simulink model "Simulacion_control"  (R2016a)
settings: Solver=ode4  SolverMode=SingleTasking  StartTime=0.0  StopTime=16  FixedStep=0.0001  RelTol=1e-3
undefined symbols (not defined in the file): ADAMS_cwd, ADAMS_exec, ADAMS_host, ADAMS_init, ADAMS_inputs, ADAMS_outputs, ADAMS_prefix, ADAMS_static, ADAMS_sysdir
libraries: simulink x5
settings Model: Creator=JoseSosa  LastModifiedBy=jrsos
settings DebuggingCC: SFUnexpectedBacktrackingDiag=error  SFNoUnconditionalDefaultTransitionDiag=error
settings SFSimCC: SimUseLocalCustomCode=on
settings RTWCC: RTWUseLocalCustomCode=on
settings GRTTargetCC: TargetLangStandard=C99 (ISO)  GeneratePreprocessorConditionals=Use local settings
settings ConfigComp: CovMetricSettings=dwe  CovHtmlReporting=off  CovSaveCumulativeToWorkspaceVar=off  CovSaveSingleToWorkspaceVar=off  CovExternalEMLEnable=on

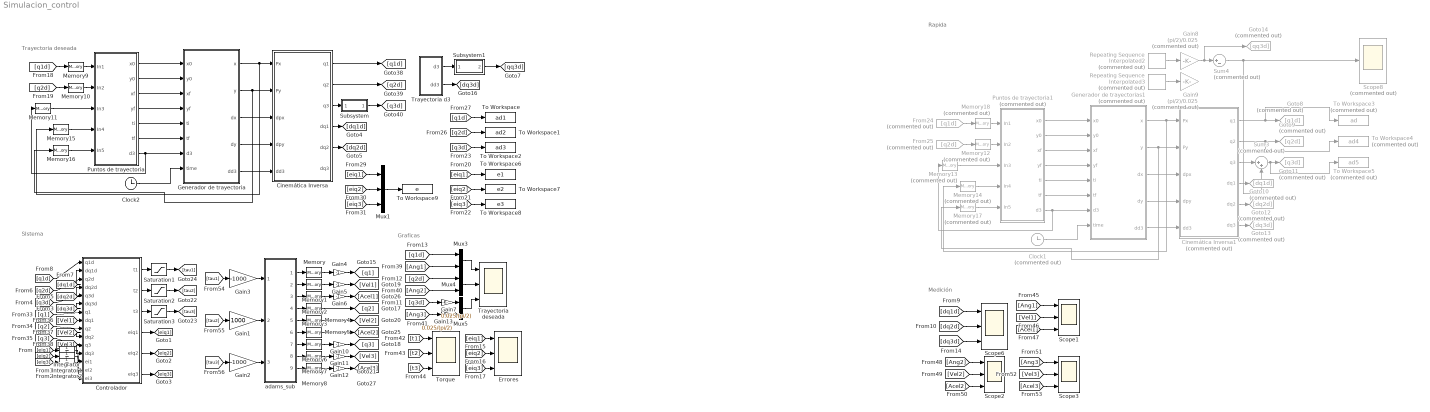
== system Simulacion_control ==
  note: Medición
  note: Graficas
  note: SIstema
  note: Trayectoria deseada
  note: Rapida
  Cinemática Inversa : MATLAB Function  TreatAsAtomicUnit=on
  Cinemática Inversa1 : MATLAB Function  Commented=on  TreatAsAtomicUnit=on
  Clock1 : Clock  Commented=on
  Clock2 : Clock
      settings: Decimation=16
  Controlador : MATLAB Function  TreatAsAtomicUnit=on
  "Errores " : Scope  NumInputPorts=3
  From24 : From  Commented=on  GotoTag=q1d
  From25 : From  Commented=on  GotoTag=q2d
  Gain1 : Gain  Gain=1000
  Gain{4..6,10..12} (6 alike) : Gain  Gain=-1
  Gain13 : Gain  Gain=0.025/(pi/2)
  Gain2 : Gain  Gain=-1000
  Gain3 : Gain  Gain=-1000
  Gain7 : Gain  Gain=0.025/(pi/2)
  Gain8 : Gain  Commented=on  Gain=(pi/2)/0.025
  Gain9 : Gain  Commented=on  Gain=(pi/2)/0.025
  Generador de trayectoria : MATLAB Function  TreatAsAtomicUnit=on
  Generador de trayectorias1 : MATLAB Function  Commented=on  TreatAsAtomicUnit=on
  Goto10 : Goto  Commented=on  GotoTag=dq1d
  Goto11 : Goto  Commented=on  GotoTag=q3d
  Goto12 : Goto  Commented=on  GotoTag=dq2d
  Goto13 : Goto  Commented=on  GotoTag=dq3d
  Goto14 : Goto  Commented=on  GotoTag=qq3d
  Goto8 : Goto  Commented=on  GotoTag=q1d
  Goto9 : Goto  Commented=on  GotoTag=q2d
  Integrator : Integrator
  Integrator1 : Integrator
  Integrator2 : Integrator
  Memory{,1..11,15..16} (14 alike) : Memory
  Memory{12..14,17..18} (5 alike) : Memory  Commented=on
  Mux1 : Mux  Inputs=3
  Mux3 : Mux  Inputs=2
  Mux4 : Mux  Inputs=2
  Mux5 : Mux  Inputs=2
  Puntos de trayectoria : Subsystem
  Puntos de trayectoria1 : Subsystem  Commented=on
  Repeating Sequence Interpolated2 : simulink/Sources/Repeating Sequence Interpolated  Commented=on  OutValues=[0 0 0.012 0.012 0 0].'  TimeValues=[0 2.9 4 6 7.1 10].'  LookUpMeth=Interpolation-Use End Values  tsamp=0.01  OutMin=[]  OutMax=[]  OutDataTypeStr=double  OutputDataTypeScalingMode=double  OutDataType=fixdt(0,8)  OutScaling=2^-10
  Repeating Sequence Interpolated3 : simulink/Sources/Repeating Sequence Interpolated  Commented=on  OutValues=[0 0 0.005 0.005 0 0].'  TimeValues=[0 4.5 5 5.5 6 10].'  LookUpMeth=Interpolation-Use End Values  tsamp=0.01  OutMin=[]  OutMax=[]  OutDataTypeStr=double  OutputDataTypeScalingMode=double  OutDataType=fixdt(0,8)  OutScaling=2^-10
  Saturation1 : Saturate  UpperLimit=6  LowerLimit=-6
  Saturation2 : Saturate  UpperLimit=6  LowerLimit=-6
  Saturation3 : Saturate  UpperLimit=6  LowerLimit=-6
  Scope{1..3,6} (4 alike) : Scope  NumInputPorts=3
  Scope8 : Scope  Commented=on
  Subsystem : Subsystem
  Subsystem1 : Subsystem
  Sum3 : Sum  Commented=on  Inputs=|++
  Sum4 : Sum  Commented=on  Inputs=|+-
  To Workspace : ToWorkspace  VariableName=ad1  SaveFormat=Timeseries  SampleTime=-1
  To Workspace1 : ToWorkspace  VariableName=ad2  SaveFormat=Timeseries  SampleTime=-1
  To Workspace2 : ToWorkspace  VariableName=ad3  SaveFormat=Timeseries  SampleTime=-1
  To Workspace3 : ToWorkspace  Commented=on  VariableName=ad  SaveFormat=Timeseries  SampleTime=-1
  To Workspace4 : ToWorkspace  Commented=on  VariableName=ad4  SaveFormat=Timeseries  SampleTime=-1
  To Workspace5 : ToWorkspace  Commented=on  VariableName=ad5  SaveFormat=Timeseries  SampleTime=-1
  To Workspace6 : ToWorkspace  VariableName=e1  SaveFormat=Timeseries  SampleTime=-1
  To Workspace7 : ToWorkspace  VariableName=e2  SaveFormat=Timeseries  SampleTime=-1
  To Workspace8 : ToWorkspace  VariableName=e3  SaveFormat=Timeseries  SampleTime=-1
  To Workspace9 : ToWorkspace  VariableName=e  SaveFormat=Timeseries  SampleTime=-1
  Torque : Scope  NumInputPorts=3
  Trayectoria d3 : Subsystem
  Trayectoria deseada : Scope  NumInputPorts=3
  adams_sub : Subsystem
  wires:
  Controlador/1(t1) -> Saturation1/1
  Controlador/3(t3) -> Saturation3/1
  Controlador/2(t2) -> Saturation2/1
  [Ang1] -> Scope1/1
  [Acel1] -> Scope1/3
  [Vel1] -> Scope1/2
  [Ang2] -> Scope2/1
  [Ang3] -> Scope3/1
  [Vel2] -> Scope2/2
  [Acel2] -> Scope2/3
  [Vel3] -> Scope3/2
  [Acel3] -> Scope3/3
  [tau1] -> Gain3/1
  [tau3] -> Gain2/1
  [tau2] -> Gain1/1
  [Vel2] -> Controlador/10(dq2)
  [q2] -> Controlador/9(q2)
  [q3] -> Controlador/11(q3)
  [Vel1] -> Controlador/8(dq1)
  [Vel3] -> Controlador/12(dq3)
  [q1] -> Controlador/7(q1)
  Memory/1 -> Gain4/1
  Gain4/1 -> [q1]
  Memory8/1 -> Gain12/1
  Memory7/1 -> Gain11/1
  Memory2/1 -> Gain6/1
  Memory1/1 -> Gain5/1
  Gain5/1 -> [Vel1]
  Gain6/1 -> [Acel1]
  Memory3/1 -> [q2]
  Memory4/1 -> [Vel2]
  Memory5/1 -> [Acel2]
  Gain10/1 -> [q3]
  Gain11/1 -> [Vel3]
  Gain12/1 -> [Acel3]
  Memory6/1 -> Gain10/1
  Mux3/1 -> Trayectoria deseada/1
  Mux4/1 -> Trayectoria deseada/2
  Mux5/1 -> Trayectoria deseada/3
  [Ang2] -> Mux4/2
  [Ang1] -> Mux3/2
  Integrator/1 -> Controlador/13(ei1)
  Integrator1/1 -> Controlador/14(ei2)
  Integrator2/1 -> Controlador/15(ei3)
  Saturation1/1 -> [tau1]
  Saturation2/1 -> [tau2]
  Saturation3/1 -> [tau3]
  Controlador/4(eiq1) -> [eiq1]
  Controlador/5(eiq2) -> [eiq2]
  Controlador/6(eiq3) -> [eiq3]
  [eiq1] -> Integrator/1
  [eiq2] -> Integrator1/1
  [eiq3] -> Integrator2/1
  [q1d] -> Controlador/1(q1d)
  [q3d] -> Controlador/5(q3d)
  [q2d] -> Controlador/3(q2d)
  [dq1d] -> Controlador/2(dq1d)
  [dq2d] -> Controlador/4(dq2d)
  [dq3d] -> Controlador/6(dq3d)
  Cinemática Inversa/1(q1) -> [q1d]
  Cinemática Inversa/2(q2) -> [q2d]
  Cinemática Inversa/4(dq1) -> [dq1d]
  Cinemática Inversa/5(dq2) -> [dq2d]
  Generador de trayectoria/2(y) -> Memory16/1, Cinemática Inversa/2(Py)
  Generador de trayectoria/1(x) -> Memory15/1, Cinemática Inversa/1(Px)
  Generador de trayectoria/3(dx) -> Cinemática Inversa/3(dpx)
  Generador de trayectoria/4(dy) -> Cinemática Inversa/4(dpy)
  [dq1d] -> Scope6/1
  [dq2d] -> Scope6/2
  [dq3d] -> Scope6/3
  Clock2/1 -> Generador de trayectoria/8(time)
  [q1d] -> Mux3/1
  [q2d] -> Mux4/1
  Generador de trayectoria/5(dd3) -> Cinemática Inversa/5(dd3)
  Puntos de trayectoria/1(x0) -> Generador de trayectoria/1(x0)
  Puntos de trayectoria/2(y0) -> Generador de trayectoria/2(y0)
  Puntos de trayectoria/3(xf) -> Generador de trayectoria/3(xf)
  Puntos de trayectoria/4(yf) -> Generador de trayectoria/4(yf)
  Puntos de trayectoria/5(ti) -> Generador de trayectoria/5(ti)
  Puntos de trayectoria/6(tf) -> Generador de trayectoria/6(tf)
  [q2d] -> Memory10/1
  [q1d] -> Memory9/1
  Memory9/1 -> Puntos de trayectoria/1(In1)
  Memory10/1 -> Puntos de trayectoria/2(In2)
  Memory11/1 -> Puntos de trayectoria/3(In3)
  Memory15/1 -> Puntos de trayectoria/4(In4)
  Memory16/1 -> Puntos de trayectoria/5(In5)
  Puntos de trayectoria/7(d3) -> Generador de trayectoria/7(d3), Memory11/1
  [eiq1] -> "Errores "/1
  [eiq2] -> "Errores "/2
  [eiq3] -> "Errores "/3
  [eiq1] -> To Workspace6/1
  [eiq2] -> To Workspace7/1
  [eiq3] -> To Workspace8/1
  Gain3/1 -> adams_sub/1(Articulacion_1.var_motor_torque)
  Gain1/1 -> adams_sub/2(Articulacion_2.var_motor_torque)
  Gain2/1 -> adams_sub/3(Articulacion_3.var_motor_torque)
  adams_sub/7(Articulacion_3.var_angdisp) -> Memory6/1
  adams_sub/8("Articulacion_3.var_omega  ") -> Memory7/1
  adams_sub/9("Articulacion_3.var_angacc ") -> Memory8/1
  adams_sub/1(Articulacion_1.var_angdisp) -> Memory/1
  adams_sub/6("Articulacion_2.var_angacc ") -> Memory5/1
  adams_sub/5("Articulacion_2.var_omega  ") -> Memory4/1
  adams_sub/4(Articulacion_2.var_angdisp) -> Memory3/1
  adams_sub/3("Articulacion_1.var_angacc ") -> Memory2/1
  adams_sub/2("Articulacion_1.var_omega  ") -> Memory1/1
  Cinemática Inversa1/1(q1) -> To Workspace3/1, Goto8/1
  Cinemática Inversa1/2(q2) -> To Workspace4/1, Goto9/1
  Cinemática Inversa1/4(dq1) -> Goto10/1
  Cinemática Inversa1/5(dq2) -> Goto12/1
  Generador de trayectorias1/2(y) -> Memory17/1, Cinemática Inversa1/2(Py)
  Generador de trayectorias1/1(x) -> Memory14/1, Cinemática Inversa1/1(Px)
  Generador de trayectorias1/3(dx) -> Cinemática Inversa1/3(dpx)
  Generador de trayectorias1/4(dy) -> Cinemática Inversa1/4(dpy)
  Cinemática Inversa1/6(dq3) -> Goto13/1
  Clock1/1 -> Generador de trayectorias1/8(time)
  Generador de trayectorias1/5(dd3) -> Cinemática Inversa1/5(dd3)
  Puntos de trayectoria1/1(x0) -> Generador de trayectorias1/1(x0)
  Puntos de trayectoria1/2(y0) -> Generador de trayectorias1/2(y0)
  Puntos de trayectoria1/3(xf) -> Generador de trayectorias1/3(xf)
  Puntos de trayectoria1/4(yf) -> Generador de trayectorias1/4(yf)
  Puntos de trayectoria1/5(ti) -> Generador de trayectorias1/5(ti)
  Puntos de trayectoria1/6(tf) -> Generador de trayectorias1/6(tf)
  From25/1 -> Memory12/1
  From24/1 -> Memory18/1
  Memory18/1 -> Puntos de trayectoria1/1(In1)
  Memory12/1 -> Puntos de trayectoria1/2(In2)
  Memory13/1 -> Puntos de trayectoria1/3(In3)
  Memory14/1 -> Puntos de trayectoria1/4(In4)
  Memory17/1 -> Puntos de trayectoria1/5(In5)
  Puntos de trayectoria1/7(d3) -> Generador de trayectorias1/7(d3), Memory13/1
  Cinemática Inversa1/3(q3) -> Sum3/1
  Repeating Sequence Interpolated2/1 -> Gain8/1
  Gain8/1 -> Sum4/1, Goto14/1
  Repeating Sequence Interpolated3/1 -> Gain9/1
  Sum4/1 -> Scope8/1, Sum3/2
  Sum3/1 -> To Workspace5/1, Goto11/1
  [t1] -> Torque/1
  [t2] -> Torque/2
  [t3] -> Torque/3
  [q3d] -> To Workspace2/1
  [q2d] -> To Workspace1/1
  [q1d] -> To Workspace/1
  Trayectoria d3/2("dd3 ") -> [dq3d]
  Subsystem1/1(2) -> [qq3d]
  Trayectoria d3/1(d3) -> Subsystem1/1(1)
  Gain7/1 -> Mux5/1
  [q3d] -> Gain7/1
  Gain13/1 -> Mux5/2
  [Ang3] -> Gain13/1
  [eiq1] -> Mux1/1
  [eiq2] -> Mux1/2
  [eiq3] -> Mux1/3
  Mux1/1 -> To Workspace9/1
  Cinemática Inversa/3(q3) -> Subsystem/1(In1)
  Subsystem/1(Out1) -> [q3d]

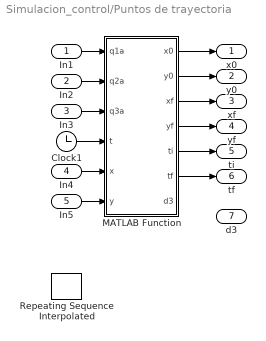
== system Simulacion_control/Puntos de trayectoria ==
  In1 : Inport
  In2 : Inport  Port=2
  In3 : Inport  Port=3
  In4 : Inport  Port=4
  In5 : Inport  Port=5
  Clock1 : Clock
      settings: Decimation=16
  MATLAB Function : MATLAB Function  TreatAsAtomicUnit=on
  Repeating Sequence Interpolated : simulink/Sources/Repeating Sequence Interpolated  OutValues=[0 0 0.015 0.015 0 0].'  TimeValues=[0 2.5 4 6 7.5 10].'  LookUpMeth=Interpolation-Use End Values  tsamp=0.01  OutMin=[]  OutMax=[]  OutDataTypeStr=double  OutputDataTypeScalingMode=double  OutDataType=fixdt(0,8)  OutScaling=2^-10
  x0 : Outport
  y0 : Outport  Port=2
  xf : Outport  Port=3
  yf : Outport  Port=4
  ti : Outport  Port=5
  tf : Outport  Port=6
  d3 : Outport  Port=7
  wires:
  Clock1/1 -> MATLAB Function/4(t)
  MATLAB Function/6(tf) -> tf/1
  MATLAB Function/1(x0) -> x0/1
  MATLAB Function/3(xf) -> xf/1
  MATLAB Function/5(ti) -> ti/1
  MATLAB Function/4(yf) -> yf/1
  MATLAB Function/2(y0) -> y0/1
  In1/1 -> MATLAB Function/1(q1a)
  In2/1 -> MATLAB Function/2(q2a)
  In3/1 -> MATLAB Function/3(q3a)
  In4/1 -> MATLAB Function/5(x)
  In5/1 -> MATLAB Function/6(y)

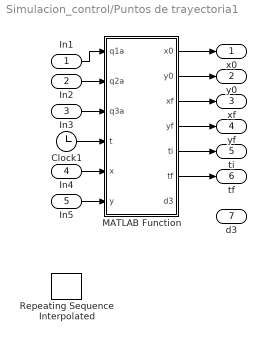
== system Simulacion_control/Puntos de trayectoria1 ==
  In1 : Inport
  In2 : Inport  Port=2
  In3 : Inport  Port=3
  In4 : Inport  Port=4
  In5 : Inport  Port=5
  Clock1 : Clock
  MATLAB Function : MATLAB Function  TreatAsAtomicUnit=on
  Repeating Sequence Interpolated : simulink/Sources/Repeating Sequence Interpolated  OutValues=[0 0 0.015 0.015 0 0].'  TimeValues=[0 2.5 4 6 7.5 10].'  LookUpMeth=Interpolation-Use End Values  tsamp=0.01  OutMin=[]  OutMax=[]  OutDataTypeStr=double  OutputDataTypeScalingMode=double  OutDataType=fixdt(0,8)  OutScaling=2^-10
  x0 : Outport
  y0 : Outport  Port=2
  xf : Outport  Port=3
  yf : Outport  Port=4
  ti : Outport  Port=5
  tf : Outport  Port=6
  d3 : Outport  Port=7
  wires:
  Clock1/1 -> MATLAB Function/4(t)
  MATLAB Function/6(tf) -> tf/1
  MATLAB Function/1(x0) -> x0/1
  MATLAB Function/3(xf) -> xf/1
  MATLAB Function/5(ti) -> ti/1
  MATLAB Function/4(yf) -> yf/1
  MATLAB Function/2(y0) -> y0/1
  In1/1 -> MATLAB Function/1(q1a)
  In2/1 -> MATLAB Function/2(q2a)
  In3/1 -> MATLAB Function/3(q3a)
  In4/1 -> MATLAB Function/5(x)
  In5/1 -> MATLAB Function/6(y)

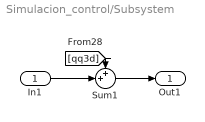
== system Simulacion_control/Subsystem ==
  In1 : Inport
  Sum1 : Sum  Inputs=++|
  Out1 : Outport
  wires:
  Sum1/1 -> Out1/1
  In1/1 -> Sum1/2
  [qq3d] -> Sum1/1

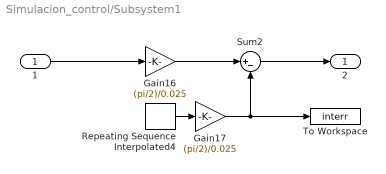
== system Simulacion_control/Subsystem1 ==
  1 : Inport
  Gain16 : Gain  Gain=(pi/2)/0.025
  Gain17 : Gain  Gain=(pi/2)/0.025
  Repeating Sequence Interpolated4 : simulink/Sources/Repeating Sequence Interpolated  OutValues=[0 0 0.005 0.005 0 0].'  TimeValues=[0 7.5 8 8.5 9 16].'  LookUpMeth=Interpolation-Use End Values  tsamp=0.01  OutMin=[]  OutMax=[]  OutDataTypeStr=double  OutputDataTypeScalingMode=double  OutDataType=fixdt(0,8)  OutScaling=2^-10
  Sum2 : Sum  Inputs=|+-
  To Workspace : ToWorkspace  VariableName=interr  SaveFormat=Structure With Time  SampleTime=-1
  2 : Outport
  wires:
  1/1 -> Gain16/1
  Sum2/1 -> 2/1
  Gain16/1 -> Sum2/1
  Repeating Sequence Interpolated4/1 -> Gain17/1
  Gain17/1 -> Sum2/2, To Workspace/1

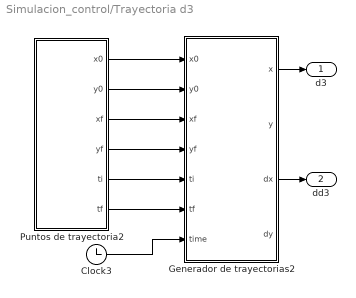
== system Simulacion_control/Trayectoria d3 ==
  Clock3 : Clock
      settings: Decimation=16
  Generador de trayectorias2 : MATLAB Function  TreatAsAtomicUnit=on
  Puntos de trayectoria2 : Subsystem
  d3 : Outport
  "dd3 " : Outport  Port=2
  wires:
  Puntos de trayectoria2/5(ti) -> Generador de trayectorias2/5(ti)
  Puntos de trayectoria2/4(yf) -> Generador de trayectorias2/4(yf)
  Generador de trayectorias2/3(dx) -> "dd3 "/1
  Generador de trayectorias2/1(x) -> d3/1
  Clock3/1 -> Generador de trayectorias2/7(time)
  Puntos de trayectoria2/6(tf) -> Generador de trayectorias2/6(tf)
  Puntos de trayectoria2/2(y0) -> Generador de trayectorias2/2(y0)
  Puntos de trayectoria2/3(xf) -> Generador de trayectorias2/3(xf)
  Puntos de trayectoria2/1(x0) -> Generador de trayectorias2/1(x0)

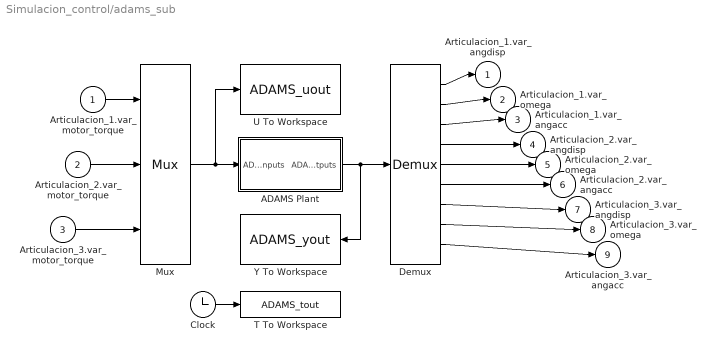
== system Simulacion_control/adams_sub ==
  Articulacion_1.var_motor_torque : Inport
  Articulacion_2.var_motor_torque : Inport  Port=2
  Articulacion_3.var_motor_torque : Inport  Port=3
  ADAMS Plant : Subsystem  LoadFcn=|  InitFcn=clear mex  mask(Adams Plant){exevie=ADAMS_sysdir, nam_in=ADAMS_inputs, namout=ADAMS_outputs, nampre=ADAMS_prefix, outfil=ADAMS_prefix, exesol=ADAMS_exec, stat=ADAMS_static, inicmd=[ADAMS_init], exetyp=C++, comtyp=PIPE(DDE), workdir=ADAMS_cwd, ada_host=ADAMS_host, modani=interactive, modsim=discrete, dft=no, simulink_lead_cosim=yes, pin_interp_order=0, pout_extrap_order=0, pin_extrap_order=0, pout_interp_order=0, dt_out=0.005, o_rate=1, more=off}
      | %check based on dialog box setting for when setting by popup menu                                             
      | if exist('ADAMS_solver_type')                                                                                 
      |   if strcmp(ADAMS_solver_type,'C++')                                                                          
      |     set_param(gcb,'exetyp','C++');                                                                            
      |   else                                                                                                        
      |     set_param(gcb,'exetyp','Fortran');                                                                        
      |   end                                                                                                         
      | else                                                                                                          
      |   set_param(gcb,'exetyp','C++');                                                                              
      | end                                                                                                           
      | %set the mode if using acar_solver                                                                            
      | %REQUIRED HERE BECAUSE BELOW CAUSES MDLTERMINATE TO BE CALLED 2 TIMES IN MIDDLE OF SIMULATION WHEN SET IN MASK
      |                                                                                                               
      | %enable the direct feedthrough, sim mode, anim mode parameters by default                                     
      |                                                                                                               
      | if exist('set_some_params_states')                                                                            
      |                                                                                                               
      |   set_some_params_states({'dft','modsim','modani'},{'on','on','on'},'MaskEnables',gcb)                        
      |   %turn on direct feedthrough option                                                                          
      |   set_some_params_states({'dft'},{'on'},'MaskVisibilities',gcb)                                               
      |                                                                                                               
      |  end                                                                                                          
      |                                                                                                               
      |                                                                                                               
      | if exist('ADAMS_exec')                                                                                        
      |   if and(strcmp(get_param(gcb,'exesol'),'ADAMS_exec'),strcmp(ADAMS_exec,'acar_solver'))                       
      |     %set the sim mode to discrete -- only supported mode                                                      
      |     set_param(gcb,'modsim','discrete')                                                                        
      |      %turn off direct feedthrough option                                                                      
      |      set_some_params_states({'dft'},{'off'},'MaskVisibilities',gcb)                                           
      |     %set the animation mode to batch -- only supported mode                                                   
      |     set_param(gcb,'modani','batch')                                                                           
      |     %disable the direct feedthrough, sim mode, anim mode parameters                                           
      |     set_some_params_states({'modsim','modani'},{'off','off'},'MaskEnables',gcb)                               
      |   end                                                                                                         
      | end
      mask prompts: exevie "Adams install directory"; nam_in "Adams View input names"; namout "Adams View output names"; nampre "Adams model file prefix"; outfil "Output files prefix (opt.: if blank - no output)"; exesol "User executable (opt.: if blank - use standard)"; stat "Initial static simulation flag"; inicmd "Initialization commands"; exetyp "Adams Solver type"; comtyp "Interprocess option"; workdir "Adams working directory"; ada_host "Adams host"; modani "Animation mode"; modsim "Simulation mode"; dft "Direct feedthrough"; simulink_lead_cosim "Discrete Computational Order - Simulink Leads Adams"; pin_interp_order "Plant input interpolation order"; pout_extrap_order "Plant output extrapolation order"; pin_extrap_order "Plant input extrapolation order"; pout_interp_order "Plant output interpolation order"; dt_out "Communication interval"; o_rate "Number of communications per output step"; more "More parameters"
      mask help: Simulate any Adams plant model either in Adams Solver form (.adm file) or in Adams View form (.cmd file)
      settings: OpenFcn=|
      | open_system(gcb,'mask')
      | if not(exist('set_some_params_states'))
      | 
      | warning('The script "set_some_params_states.m" cannot be found in the MATLAB PATH.  Cannot update the ADAMS Plant S-Function parameters.')
      | 
      | warning('Recommended action(optional):  run the Adams Controls .m file first to help choose the correct settings in the Adams S-Function block.')
      | 
      | end
      mask Help:
      | <html>
      | This S-Function represents the non-linear Adams Plant with the inputs sent to the Adams model <br>
      |  and the outputs generated by the Adams model.  See the Adams Controls documentation for more <br>
      | information.  This plant uses the following variables:<br>
      | <br>
      | <b>ADAMS_sysdir  :</b> Adams installation directory<br>
      | <b>ADAMS_inputs  :</b> Input variables View names vector<br>
      | <b>ADAMS_outputs :</b> Outputs variables View names vector<br>
      | <b>ADAMS_prefix  : </b>ADAMS model files prefix (.adm, .cmd); also doubles as output files prefix<br>
      | <b>ADAMS_exec :</b> Adams Solver user library or keyword (e.g., acar_solver)<br>
      | <b>ADAMS_static :</b> yes|no - initial static before Co-simulation(discrete)/Function Evaluation(continuous)<br>
      | <b>ADAMS_init :</b>Initialization commands (i.e., Adams View or Solver commands, depending on setting for Animation mode)<br>
      | <b>ADAMS_cwd : </b> Current working directory (for TCP/IP)<br>
      | <b>ADAMS_host : </b>Name of Adams server host (for TCP/IP)<br>
      | <b>ADAMS_mode :</b> Linear or non-linear (i.e., co-sim, function eval)<br>
      | <b>ADAMS_solver_type :</b>Fortran or C++ (used to set popup menu when first loaded) <br>
      | 
      | 
      | <br>
      | The following settings can be chosen:<br>
      | <br>
      | <b>Adams Solver type:</b>  Fortran or C++ (will also set ADAMS_solver_type)<br>
      | <b>Interprocess option:</b> Pipe(DDE) or TCP/IP; TCP/IP can allow different machines run Adams and MATLAB<br>
      | <b>Animation mode:</b> batch (Solver, uses .adm) or interactive (View, uses .cmd)<br>
      | <b>Simulation mode:</b> discrete (Co-simulation) or continuous (Function Evaluation)<br>
      | <b>Discrete Computational Order - Simulink Lead Adams:</b> for discrete mode, chooses if Simulink leads the integration (yes) or lags (no);<br> if set to "no", can remove algebraic loop<br>
      | <b>Plant input interpolation order:</b> 0 = zero-order hold; 1 = linear (discrete mode only, where Simulink leads)<br>
      | <b>Plant output extrapolation order:</b> 0 = zero-order hold;1 = linear(discrete mode only, where Simulink leads)<br>
      | <b>Plant input extrapolation order:</b> 0 = zero-order hold; 1 = linear (discrete mode only, where Adams leads)<br>
      | <b>Plant output interpolation order:</b> 0 = zero-order hold;1 = linear(discrete mode only, where Adams leads)<br>
      | <b>Direct feedthrough:</b> yes|no - yes = Input directly effect output(continuous mode-only)<br>
      | <b>Communication interval:</b> Time step at which Co-simulation exchange information (e.g.,0.005); also controls <br>output for continuous mode (Function Evaluation)<br>
      | <b>Number of communications per output step: </b>Sets Adams output rate (.res, .req, .gra) integer value (default: 1)<br>
      | </html>
      mask Callback exesol:
      | if exist('set_some_params_states')
      | %enable the direct feedthrough, sim mode, anim mode parameters
      | set_some_params_states({'dft','modsim','modani'},{'on','on','on'},'MaskEnables',gcb)
      | %turn on direct feedthrough option
      | set_some_params_states({'dft'},{'on'},'MaskVisibilities',gcb)
      | end
      | 
      | if exist('ADAMS_exec')
      |   if and(strcmp(get_param(gcb,'exesol'),'ADAMS_exec'),strcmp(ADAMS_exec,'acar_solver'))
      |     %set the sim mode to discrete -- only supported mode
      |     %REMOVED:  BELOW CAUSES MDLTERMINATE TO BE CALLED 2 TIMES IN MIDDLE OF SIMULATION
      |     %Now in LoadFcn callback
      |     %set_param(gcb,'modsim','discrete')
      |      %turn off direct feedthrough option
      |     set_some_params_states({'dft'},{'off'},'MaskVisibilities',gcb)
      |     %set the animation mode to batch -- only supported mode
      |     %REMOVED:  BELOW CAUSES MDLTERMINATE TO BE CALLED 2 TIMES IN MIDDLE OF SIMULATION
      |     %Now in LoadFcn callback
      |     %set_param(gcb,'modani','batch')
      |     %disable the direct feedthrough, sim mode, anim mode parameters
      |     set_some_params_states({'modsim','modani'},{'off','off'},'MaskEnables',gcb)
      |   end
      | end
      mask TypeOptions exetyp: Fortran | C++
      mask Callback exetyp:
      | if strcmp(get_param(gcb,'exetyp'),'C++')
      |     ADAMS_solver_type='C++';
      | else
      |     ADAMS_solver_type='Fortran';
      | end
      mask TypeOptions comtyp: PIPE(DDE) | TCP/IP
      mask Callback comtyp:
      | if exist('set_some_params_states')
      | if strcmp(get_param(gcb,'comtyp'),'PIPE(DDE)')
      |     %turn off cwd, host options
      |     set_some_params_states({'ada_host','workdir'},{'off','off'},'MaskVisibilities',gcb)
      | else%if strcmp(get_param(gcb,'modsim'),'TCP/IP')
      |     %turn on cwd, host options
      |     set_some_params_states({'ada_host','workdir'},{'on','on'},'MaskVisibilities',gcb)
      | end
      | end
      mask TypeOptions modani: batch | interactive
      mask TypeOptions modsim: discrete | continuous
      mask Callback modsim:
      | if exist('set_some_params_states')
      | if strcmp(get_param(gcb,'modsim'),'discrete')
      |      %turn off direct feedthrough option
      |     set_some_params_states({'dft'},{'off'},'MaskVisibilities',gcb)
      |     %turn on discrete co-sim type if want to see more
      |     if strcmp(get_param(gcb,'more'),'on')
      |         set_some_params_states({'simulink_lead_cosim'},{'on'},'MaskVisibilities',gcb)
      |     end
      |     if strcmp(get_param(gcb,'simulink_lead_cosim'),'yes')
      |         %turn on interpolation/extrapolation options
      |         set_some_params_states({'pin_interp_order','pout_extrap_order',},{'on','on'},'MaskVisibilities',gcb)
      |     else
      |         set_some_params_states({'pin_extrap_order','pout_interp_order'},{'on','on'},'MaskVisibilities',gcb)
      |     end
      | else%if strcmp(get_param(gcb,'modsim'),'continuous')
      |      %turn off direct feedthrough option
      |     set_some_params_states({'dft'},{'on'},'MaskVisibilities',gcb)
      |     %turn off interpolation/extrapolation options
      |     set_some_params_states({'pin_interp_order','pout_extrap_order','pin_extrap_order','pout_interp_order','simulink_lead_cosim'},{'off','off','off','off','off'},'MaskVisibilities',gcb)
      | end
      | end
      mask TypeOptions dft: no | yes
      mask TypeOptions simulink_lead_cosim: yes | no
      mask Callback simulink_lead_cosim:
      | if exist('set_some_params_states')
      | if (strcmp(get_param(gcb,'simulink_lead_cosim'),'yes') && strcmp(get_param(gcb,'modsim'),'discrete'))
      |      %turn off unused interpolate/extrapolate options
      |     set_some_params_states({'pin_extrap_order','pout_interp_order'},{'off','off'},'MaskVisibilities',gcb)
      |     %turn on used interpolate/extrapolate options
      |     set_some_params_states({'pin_interp_order','pout_extrap_order'},{'on','on'},'MaskVisibilities',gcb)
      | elseif (strcmp(get_param(gcb,'simulink_lead_cosim'),'no') && strcmp(get_param(gcb,'modsim'),'discrete'))
      |     %turn on used interpolate/extrapolate options
      |     set_some_params_states({'pin_extrap_order','pout_interp_order'},{'on','on'},'MaskVisibilities',gcb)
      |      %turn off unused interpolate/extrapolate options
      |     set_some_params_states({'pin_interp_order','pout_extrap_order'},{'off','off'},'MaskVisibilities',gcb)
      | end
      | end
      mask TypeOptions pin_interp_order: 0 | 1
      mask TypeOptions pout_extrap_order: 0 | 1
      mask TypeOptions pin_extrap_order: 0 | 1
      mask TypeOptions pout_interp_order: 0 | 1
      mask Callback more:
      | if exist('set_some_params_states')
      | if (strcmp(get_param(gcb,'more'),'on'))
      |      %turn on infrequently used options
      |     set_some_params_states({'exevie','nam_in','namout','exesol','stat','inicmd'},{'on','on','on','on','on','on'},'MaskVisibilities',gcb)
      |     if strcmp(get_param(gcb,'modsim'),'discrete')
      |         set_some_params_states({'simulink_lead_cosim'},{'on'},'MaskVisibilities',gcb)
      |     end
      | elseif (strcmp(get_param(gcb,'more'),'off'))
      |     %turn off infrequently used options
      |     set_some_params_states({'exevie','nam_in','namout','exesol','stat','inicmd'},{'off','off','off','off','off','off'},'MaskVisibilities',gcb)
      |     if strcmp(get_param(gcb,'modsim'),'discrete')
      |         set_some_params_states({'simulink_lead_cosim'},{'off'},'MaskVisibilities',gcb)
      |     end
      | end
      | end
      mask Display: disp( 'MSC Software' )
  Clock : Clock
  Demux : Demux  Outputs=9
  Mux : Mux  Inputs=3
  T To Workspace : ToWorkspace  VariableName=ADAMS_tout
      settings: MaxDataPoints=100000
  U To Workspace : ToWorkspace  VariableName=ADAMS_uout
      settings: MaxDataPoints=100000
  Y To Workspace : ToWorkspace  VariableName=ADAMS_yout
      settings: MaxDataPoints=160000
  Articulacion_1.var_angdisp : Outport
  "Articulacion_1.var_omega  " : Outport  Port=2
  "Articulacion_1.var_angacc " : Outport  Port=3
  Articulacion_2.var_angdisp : Outport  Port=4
  "Articulacion_2.var_omega  " : Outport  Port=5
  "Articulacion_2.var_angacc " : Outport  Port=6
  Articulacion_3.var_angdisp : Outport  Port=7
  "Articulacion_3.var_omega  " : Outport  Port=8
  "Articulacion_3.var_angacc " : Outport  Port=9
  wires:
  Clock/1 -> T To Workspace/1
  Mux/1 -> ADAMS Plant/1(ADAMS inputs), U To Workspace/1
  ADAMS Plant/1(ADAMS outputs) -> Demux/1, Y To Workspace/1
  Demux/1 -> Articulacion_1.var_angdisp/1
  Demux/2 -> "Articulacion_1.var_omega  "/1
  Demux/3 -> "Articulacion_1.var_angacc "/1
  Demux/4 -> Articulacion_2.var_angdisp/1
  Demux/5 -> "Articulacion_2.var_omega  "/1
  Demux/6 -> "Articulacion_2.var_angacc "/1
  Demux/7 -> Articulacion_3.var_angdisp/1
  Demux/8 -> "Articulacion_3.var_omega  "/1
  Demux/9 -> "Articulacion_3.var_angacc "/1
  Articulacion_1.var_motor_torque/1 -> Mux/1
  Articulacion_2.var_motor_torque/1 -> Mux/2
  Articulacion_3.var_motor_torque/1 -> Mux/3

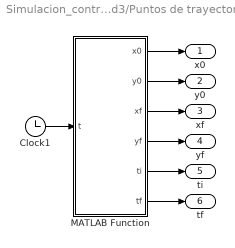
== system Simulacion_control/Trayectoria d3/Puntos de trayectoria2 ==
  Clock1 : Clock
      settings: Decimation=16
  MATLAB Function : MATLAB Function  TreatAsAtomicUnit=on
  x0 : Outport
  y0 : Outport  Port=2
  xf : Outport  Port=3
  yf : Outport  Port=4
  ti : Outport  Port=5
  tf : Outport  Port=6
  wires:
  Clock1/1 -> MATLAB Function/1(t)
  MATLAB Function/1(x0) -> x0/1
  MATLAB Function/2(y0) -> y0/1
  MATLAB Function/3(xf) -> xf/1
  MATLAB Function/4(yf) -> yf/1
  MATLAB Function/5(ti) -> ti/1
  MATLAB Function/6(tf) -> tf/1

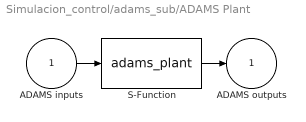
== system Simulacion_control/adams_sub/ADAMS Plant ==
  ADAMS inputs : Inport
  S-Function : S-Function  StopFcn=clear mex  FunctionName=adams_plant  Parameters=exevie,exesol,stat,outfil,nampre,o_rate,nam_in,namout,dft,modsim,modani,dt_out,inicmd,exetyp,comtyp,ada_host, workdir,pin_interp_order,pout_extrap_order,pin_extrap_order,pout_interp_order,simulink_lead_cosim  SFunctionDeploymentMode=off  EnableBusSupport=off
  ADAMS outputs : Outport  InitialOutput=0
  wires:
  ADAMS inputs/1 -> S-Function/1
  S-Function/1 -> ADAMS outputs/1

== matlab function Simulacion_control/Generador de trayectoria ==
  data: x output; x0 input; y output; y0 input; xf input; yf input; ti input; tf input; d3 input; dx output; dy output; time input; dd3 output
function [x,y,dx,dy,dd3]= Gen_trayec(x0,y0,xf,yf,ti,tf,d3,time)
t0=ti;
t_int=tf;
t=time-t0;
difx=xf-x0;
if(t >=t_int)
    t=tf;
end
if(difx==0)
    difx=0.000001;
end

m=(yf-y0)/(difx);
b=y0-m*x0;

%Coeficientes cúbicos para la coordenada x 
ax0=x0;
ax1=0;
ax2=(3/(tf*tf))*(difx);
ax3=(-2/(tf*tf*tf))*(difx);
%Movimiento para la cordenada x con polinomio cúbico
x=ax0+ax1*t+ax2*t*t+ax3*t*t*t;
dx=ax1+2*ax2*t+3*ax3*t*t;

%Movimiento para coordenada y
y=m*x+b;
dy=m*dx;

dd3=d3;

== matlab function Simulacion_control/Puntos de trayectoria/MATLAB Function ==
  data: q1a input; q2a input; q3a input; x0 output; y0 output; xf output; yf output; ti output; tf output; t input; d3 output; x input; y input
function [x0,y0, xf,yf,ti,tf,d3] = fcn(q1a,q2a,q3a,t,x,y)
L1 = .42;
L2 = .14;
L3 = .305;
x0 = 0;
y0 = 0;
xf = 0;
yf = 0;
tf  = 0;
ti = 0;
d3=0;
if t<=2.5
    x0 = 0.28;
    y0 = 0.305;
    xf = 0.1187;%0.42;
    yf = 0.2920;%0.445;
    tf  = 2.5;
    ti = 0;
    d3=0;
% else
%     q3a;
%     px = L1 + L3*cos(q1a + q2a - (pi/2)) + q3a*cos(q1a + q2a - (pi/2)) - L2*cos(q1a);
%     py = L2*sin(q1a) - q3a*sin(q1a + q2a - (pi/2)) - L3*sin(q1a + q2a - (pi/2));
%     x0 = x;
%     y0 = y;
%     xf = px%0.1187;%0.42;
%     yf = py%0.2920;%0.445;
%     tf  = 2.5;
%     ti = 0;
%     d3=0;


elseif t<=7
    x0 = 0.1187;%0.42;
    y0 = 0.2920; %0.445;
    xf = 0.1187;%0.42;
    yf = 0.2920; %0.445;
%     xf = 0.1105;%0.42;
%     yf = 0.3046;%0.445;
    tf  = 4.5;
    ti = 2.5;
    d3=0.015;
elseif t<=9
    x0 = 0.1187;%0.42;
    y0 = 0.2920; %0.445;
    xf = 0.1187;%0.42;
    yf = 0.2920; %0.445;
%     x0 = 0.1105;%0.42;
%     y0 = 0.3046;%0.445;
%     xf = 0.1105;%0.42;
%     yf = 0.3046;%0.445;
    tf  = 2;
    ti = 7;
    d3=0.015;
elseif t<=13.5
    x0 = 0.1187;%0.42;
    y0 = 0.2920; %0.445;
    xf = 0.1187;%0.42;
    yf = 0.2920; %0.445;
%     x0 = 0.1105;%0.42;
%     y0 = 0.3046;%0.445;
%     xf = 0.1187;%0.42;
%     yf = 0.2920;%0.445;
    tf  = 4.5;
    ti = 9;
    d3=0;
elseif t<=16
    x0 = 0.1187;%0.42;
    y0 = 0.2920;%0.445;
    xf = 0.28;
    yf = 0.305;
    tf  = 2.5;
    ti = 13.5;
    d3=0;
end

== matlab function Simulacion_control/Cinemática Inversa ==
  data: Px input; q1 output; q2 output; q3 output; Py input; dpx input; dpy input; dd3 input; dq1 output; dq2 output; dq3 output
function [q1,q2,q3,dq1,dq2,dq3]= cinematica(Px,Py,dpx,dpy,dd3)
if dd3 >= 0.025
    dd3 = 0.025;
end
if dd3 <= 0
    dd3 = 0;
end
H1 =  0.42;
L1 = 0.14;
L2 = 0.305;
L3 = L2 + dd3;

Px1 = H1 - Px;
r1_2 = Px1^2 + Py^2;
r1 = sqrt(r1_2);

M = (r1_2 - L1^2 - L3^2)/(2*L1*L3);
if M >= 1
    M = 1;
end
if M <= -1
    M = -1;
end

th2 = atan2d(sqrt(1-M^2),M)-90;

M2 = (r1_2 + L1^2 - L3^2)/(2*L1*r1);
if M2 >= 1
    M2 = 1;
end
if M2 <= -1
    M2 = -1;    
end

b2 = atan2d(sqrt(1-M2^2),M2);

% if Py/Px1 <= 1.5 && Py/Px1 >= -0.01 
%     b1 = 360+atan2d(Py,Px1);
%     th1 = b1 - b2;
% else
    th1 = atan2d(Py,Px1) - b2;
% end
% th1 = atan2d(Py,Px1) - acosd(M2)
%dd3 = dd3*90/0.03;
d3=dd3*(pi/2)/0.025;
th1=th1*pi/180;
th2=th2*pi/180;

q1 = th1;
q2 = th2;
q3 = d3;
%% Jacobiano inverso
lc3=0.093;
q1 = th1;
q2 = th2;
q3 = d3;
L1=0.14;
L2=0.305;

J3 = [ L2*cos(q1 + q2) + L1*sin(q1) + cos(q1 + q2)*(q3 - lc3), cos(q1 + q2)*(L2 + q3 - lc3), sin(q1 + q2);
          L1*cos(q1) - L2*sin(q1 + q2) - sin(q1 + q2)*(q3 - lc3), -sin(q1 + q2)*(L2 + q3 - lc3), cos(q1 + q2);
          0,  0, 0];

velCar = [dpx; dpy];
      
J = [J3(1,1:3); J3(2,1:3)];
JT = [J(1,1) J(2,1); J(1,2) J(2,2); J(1,3) J(2,3)];

JJ = J*JT;
iJJ = inv(JJ);
pinJ = JT*iJJ;
pinJ = pinJ*velCar;
dq1 = pinJ(1);
dq2 = pinJ(2);
dq3 = pinJ(3);

== matlab function Simulacion_control/Cinemática Inversa1 ==
  data: Px input; q1 output; q2 output; q3 output; Py input; dpx input; dpy input; dd3 input; dq1 output; dq2 output; dq3 output
function [q1,q2,q3,dq1,dq2,dq3]= cinematica(Px,Py,dpx,dpy,dd3)
if dd3 >= 0.025
    dd3 = 0.025;
end
if dd3 <= 0
    dd3 = 0;
end
H1 =  0.42;
L1 = 0.14;
L2 = 0.305;
L3 = L2 + dd3;

Px1 = H1 - Px;
r1_2 = Px1^2 + Py^2;
r1 = sqrt(r1_2);

M = (r1_2 - L1^2 - L3^2)/(2*L1*L3);
if M >= 1
    M = 1;
end
if M <= -1
    M = -1;
end

th2 = atan2d(sqrt(1-M^2),M)-90;

M2 = (r1_2 + L1^2 - L3^2)/(2*L1*r1);
if M2 >= 1
    M2 = 1;
end
if M2 <= -1
    M2 = -1;    
end

b2 = atan2d(sqrt(1-M2^2),M2);

% if Py/Px1 <= 1.5 && Py/Px1 >= -0.01 
%     b1 = 360+atan2d(Py,Px1);
%     th1 = b1 - b2;
% else
    th1 = atan2d(Py,Px1) - b2;
% end
% th1 = atan2d(Py,Px1) - acosd(M2)
%dd3 = dd3*90/0.03;
d3=dd3*(pi/2)/0.025;
th1=th1*pi/180;
th2=th2*pi/180;

q1 = th1;
q2 = th2;
q3 = d3;
%% Jacobiano inverso
lc3=0.093;
q1 = th1;
q2 = th2;
q3 = d3;
L1=0.14;
L2=0.305;

J3 = [ L2*cos(q1 + q2) + L1*sin(q1) + cos(q1 + q2)*(q3 - lc3), cos(q1 + q2)*(L2 + q3 - lc3), sin(q1 + q2);
          L1*cos(q1) - L2*sin(q1 + q2) - sin(q1 + q2)*(q3 - lc3), -sin(q1 + q2)*(L2 + q3 - lc3), cos(q1 + q2);
          0,  0, 0];

velCar = [dpx; dpy];
      
J = [J3(1,1:3); J3(2,1:3)];
JT = [J(1,1) J(2,1); J(1,2) J(2,2); J(1,3) J(2,3)];

JJ = J*JT;
iJJ = inv(JJ);
pinJ = JT*iJJ;
pinJ = pinJ*velCar;
dq1 = pinJ(1);
dq2 = pinJ(2);
dq3 = pinJ(3);

== matlab function Simulacion_control/Controlador ==
  data: q1d input; t1 output; t2 output; t3 output; dq1d input; q2d input; dq2d input; q3d input; dq3d input; q1 input; dq1 input; q2 input; dq2 input; q3 input; dq3 input; eiq1 output; ei1 input; ei2 input; ei3 input; eiq2 output; eiq3 output
function [t1,t2,t3, eiq1, eiq2, eiq3]= Controlador(q1d,dq1d,q2d,dq2d,q3d,dq3d,q1,dq1,q2,dq2,q3,dq3,ei1,ei2,ei3)
%NOTA: q1, q2 y q3 en radianes
%% Parametros del sistema
L1=0.14;
L2=0.305;

lc1=0.21;
lc2=0.164448 + (q3/2)*0.025/(pi/2);
lc3=0.093;

m1 = 0.3642;
m2 = 0.767;
m3 = 0.0044;
g=-9.81;
%% errores
eq1=q1d-q1;
eq2=q2d-q2;
eq3=q3d-q3;

deq1=dq1d-dq1;
deq2=dq2d-dq2;
deq3=dq3d-dq3;
%% Ganancias
kp1=12;
kp2=7;
kp3=0.3;

kv1=0.07*kp1;
kv2=0.06*kp2;
kv3=0.02*kp3;
% kv1=0.07*kp1;
% kv2=0.06*kp2;
% kv3=0.02*kp3;

ki1=4.5*kp1;
ki2=4*kp2;
ki3=3*kp3;
% ki1=4.5*kp1;
% ki2=4*kp2;
% ki3=3*kp3;
%% Matrices de error y ganancias
Kp=[kp1 0 0;0 kp2 0;0 0 kp3];
Kv=[kv1 0 0;0 kv2 0;0 0 kv3];
Ki=[ki1 0 0;0 ki2 0;0 0 ki3];

eq=[eq1; eq2;eq3];
deq=[deq1;deq2;deq3];
ei=[ei1;ei2;ei3];
%% Salidas del integrador
eiq1 = eq1;
eiq2 = eq2;
eiq3 = eq3;
%% Vector de gravedad
g1 = -g*m3*(L1*sin(q1)+L2*cos(q1 + q2)+(lc3 + q3)*cos(q1 + q2))-g*m2*(lc2*cos(q1 + q2) + L1*sin(q1))-g*lc1*m1*sin(q1);
g2 = -g*m3*(L2*cos(q1 + q2)+(lc3 + q3)*cos(q1 + q2))-g*cos(q1 + q2)*lc2*m2;
g3 = -m3*g*sin(q1 + q2);
gq=[g1; g2; g3];
%% Control PD+g
T=Kp*eq+Kv*deq+Ki*ei+gq;
t1=T(1);
t2=T(2);
t3=T(3);

== matlab function Simulacion_control/Generador de trayectorias1 ==
  data: x output; x0 input; y output; y0 input; xf input; yf input; ti input; tf input; d3 input; dx output; dy output; time input; dd3 output
function [x,y,dx,dy,dd3]= Gen_trayec(x0,y0,xf,yf,ti,tf,d3,time)
t0=ti;
t_int=tf;
t=time-t0;
difx=xf-x0;
if(t >=t_int)
    t=tf;
end
if(difx==0)
    difx=0.000001;
end

m=(yf-y0)/(difx);
b=y0-m*x0;

%Coeficientes cúbicos para la coordenada x 
ax0=x0;
ax1=0;
ax2=(3/(tf*tf))*(difx);
ax3=(-2/(tf*tf*tf))*(difx);
%Movimiento para la cordenada x con polinomio cúbico
x=ax0+ax1*t+ax2*t*t+ax3*t*t*t;
dx=ax1+2*ax2*t+3*ax3*t*t;

%Movimiento para coordenada y
y=m*x+b;
dy=m*dx;

dd3=d3;

== matlab function Simulacion_control/Puntos de trayectoria1/MATLAB Function ==
  data: q1a input; q2a input; q3a input; x0 output; y0 output; xf output; yf output; ti output; tf output; t input; d3 output; x input; y input
function [x0,y0, xf,yf,ti,tf,d3] = fcn(q1a,q2a,q3a,t,x,y)
L1 = .42;
L2 = .14;
L3 = .305;
x0 = 0;
y0 = 0;
xf = 0;
yf = 0;
tf  = 0;
ti = 0;
d3=0;
if t<=2.5
    x0 = 0.28;
    y0 = 0.305;
    xf = 0.1187;%0.42;
    yf = 0.2920;%0.445;
    tf  = 2.5;
    ti = 0;
    d3=0;
% else
%     q3a;
%     px = L1 + L3*cos(q1a + q2a - (pi/2)) + q3a*cos(q1a + q2a - (pi/2)) - L2*cos(q1a);
%     py = L2*sin(q1a) - q3a*sin(q1a + q2a - (pi/2)) - L3*sin(q1a + q2a - (pi/2));
%     x0 = x;
%     y0 = y;
%     xf = px%0.1187;%0.42;
%     yf = py%0.2920;%0.445;
%     tf  = 2.5;
%     ti = 0;
%     d3=0;


elseif t<=4
    x0 = 0.1187;%0.42;
    y0 = 0.2920; %0.445;
    xf = 0.1187;%0.42;
    yf = 0.2920; %0.445;
%     xf = 0.1105;%0.42;
%     yf = 0.3046;%0.445;
    tf  = 1.5;
    ti = 2.5;
    d3=0.015;
elseif t<=6
    x0 = 0.1187;%0.42;
    y0 = 0.2920; %0.445;
    xf = 0.1187;%0.42;
    yf = 0.2920; %0.445;
%     x0 = 0.1105;%0.42;
%     y0 = 0.3046;%0.445;
%     xf = 0.1105;%0.42;
%     yf = 0.3046;%0.445;
    tf  = 2;
    ti = 4;
    d3=0.015;
elseif t<=7.5
    x0 = 0.1187;%0.42;
    y0 = 0.2920; %0.445;
    xf = 0.1187;%0.42;
    yf = 0.2920; %0.445;
%     x0 = 0.1105;%0.42;
%     y0 = 0.3046;%0.445;
%     xf = 0.1187;%0.42;
%     yf = 0.2920;%0.445;
    tf  = 1.5;
    ti = 6;
    d3=0;
elseif t<=10
    x0 = 0.1187;%0.42;
    y0 = 0.2920;%0.445;
    xf = 0.28;
    yf = 0.305;
    tf  = 2.5;
    ti = 7.5;
    d3=0;
end

== matlab function Simulacion_control/Trayectoria d3/Puntos de trayectoria2/MATLAB Function ==
  data: t input; x0 output; y0 output; xf output; yf output; ti output; tf output
function [x0,y0, xf,yf,ti,tf] = fcn(t)
x0 = 0;
y0 = 0;
xf = 0;
yf = 0;
tf  = 0;
ti = 0;
d3=0;
if t<=5
    x0 = 0;
    y0 = 0;
    xf = 0;
    yf = 0;
    tf  = 7;
    ti = 0;
elseif t<=7
    x0 = 0;
    y0 = 0;
    xf = 0.012;
    yf = 0;
    tf  = 2;
    ti = 5;
elseif t<=9
    x0 = 0.012;
    y0 = 0;
    xf = 0.012;
    yf = 0;
    tf  = 2;
    ti = 7;
elseif t<=11
    x0 = 0.012;
    y0 = 0;
    xf = 0;
    yf = 0;
    tf  = 2;
    ti = 9;
elseif t<=16
    x0 = 0;
    y0 = 0;
    xf = 0;
    yf = 0;
    tf  = 5;
    ti = 11;
end

== matlab function Simulacion_control/Trayectoria d3/Generador de trayectorias2 ==
  data: x output; x0 input; y output; y0 input; xf input; yf input; ti input; tf input; dx output; dy output; time input
function [x,y,dx,dy]= Gen_trayec(x0,y0,xf,yf,ti,tf,time)
t0=ti;
t_int=tf;
t=time-t0;
difx=xf-x0;
if(t >=t_int)
    t=tf;
end
if(difx==0)
    difx=0.000001;
end

m=(yf-y0)/(difx);
b=y0-m*x0;

%Coeficientes cúbicos para la coordenada x 
ax0=x0;
ax1=0;
ax2=(3/(tf*tf))*(difx);
ax3=(-2/(tf*tf*tf))*(difx);
%Movimiento para la cordenada x con polinomio cúbico
x=ax0+ax1*t+ax2*t*t+ax3*t*t*t;
dx=ax1+2*ax2*t+3*ax3*t*t;

%Movimiento para coordenada y
y=m*x+b;
dy=m*dx;
